simulink model "IntroductiontoSubsystems"  (R2025a)
settings: Solver=VariableStepAuto  StartTime=0.0  StopTime=10.0  RelTol=1e-3
model workspace (MAT data in the model file):
  Ts = 0.01
  ki = 7.33
  kp = 9.39
undefined symbols (not defined in the file or in its folder): b, J, K, L, R, V
libraries: SignalEditorBlockLib x1
settings Model: Creator=JPIRES3  LastModifiedBy=JPIRES3

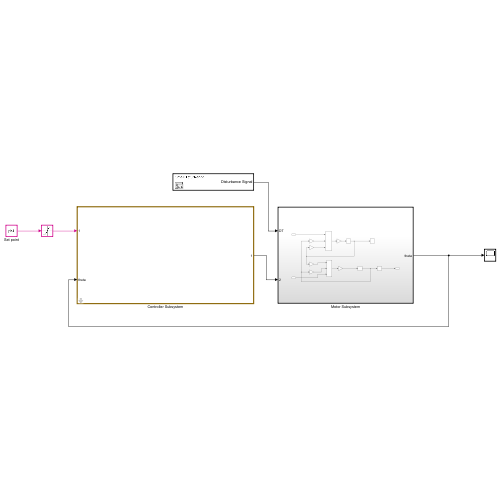
[thumbnail: Simulink's stored preview of the top-level diagram]
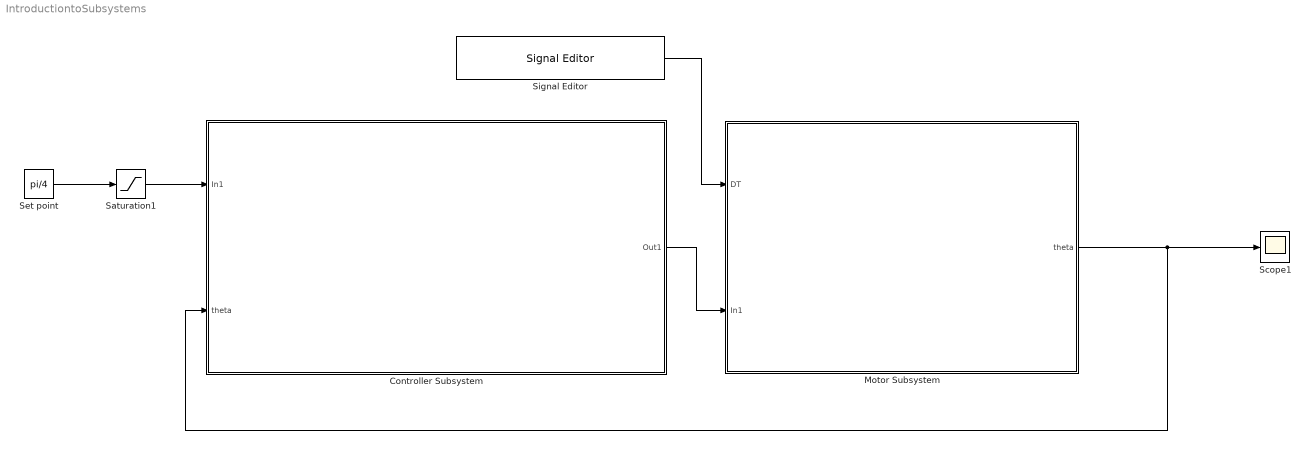
== system IntroductiontoSubsystems ==
  Controller Subsystem : Subsystem  TreatAsAtomicUnit=on  mask{kp=9.39, ki=7.33, Ts=0.01}
      mask prompts: kp "proportional Gain"; ki "Integral Gain"; Ts "Sample Time"
  Motor Subsystem : Subsystem
  Saturation1 : Saturate  UpperLimit=pi/4  LowerLimit=-pi/4
  Scope1 : Scope
      settings: ActiveDisplayYMinimum=-0.11554258584712604  ActiveDisplayYMaximum=1.0398832726241345
  Set point : Constant  Value=pi/4
  Signal Editor : SignalEditorBlockLib/Signal Editor  FileName=C:\Users\jpires3\Documents\Matlab-projects\Module 3 - Introduction to subsystems\Disturbance.mat  ActiveScenario=SmallDisturbance  ActiveSignal=Disturbance Signal  IsBus=off  OutputBusObjectStr=Bus: BusObject  SampleTime=0  ZeroCross=off  OutputAfterFinalValue=Setting to zero  Unit=inherit  PreserveSignalName=on  ApplySigPropsToAllScenarios=on  ApplySigPropsToAllSignals=off  SignalPropertySource=Dialog parameters
  wires:
  Set point/1 -> Saturation1/1
  Motor Subsystem/1(theta) -> Controller Subsystem/2(theta), Scope1/1
  Saturation1/1 -> Controller Subsystem/1(In1)
  Controller Subsystem/1(Out1) -> Motor Subsystem/2(In1)
  Signal Editor/1 -> Motor Subsystem/1(DT)

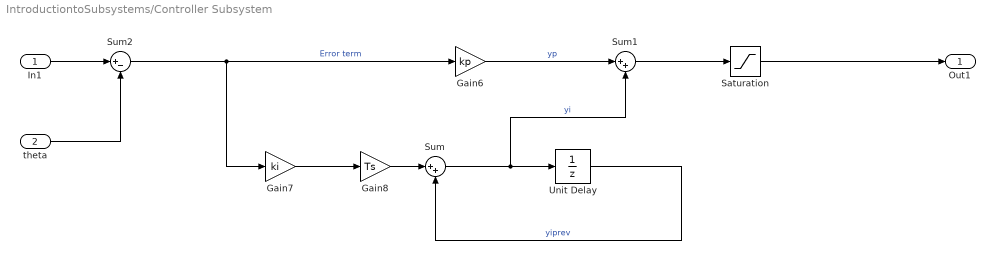
== system IntroductiontoSubsystems/Controller Subsystem ==
  In1 : Inport
  theta : Inport  Port=2
  Gain6 : Gain  Gain=kp
  Gain7 : Gain  Gain=ki
  Gain8 : Gain  Gain=Ts
  Saturation : Saturate  UpperLimit=V  LowerLimit=-V
  Sum : Sum  Inputs=|++
  Sum1 : Sum  Inputs=|++
  Sum2 : Sum  Inputs=|+-
  Unit Delay : UnitDelay  InitialCondition=1  SampleTime=Ts  HasFrameUpgradeWarning=on
  Out1 : Outport
  wires:
  Gain8/1 -> Sum/1
  Sum/1 -> Sum1/2, Unit Delay/1  "yi"
  Sum1/1 -> Saturation/1
  Unit Delay/1 -> Sum/2  "yiprev"
  In1/1 -> Sum2/1
  Gain6/1 -> Sum1/1  "yp"
  Sum2/1 -> Gain7/1, Gain6/1  "Error term"
  Saturation/1 -> Out1/1
  Gain7/1 -> Gain8/1
  theta/1 -> Sum2/2

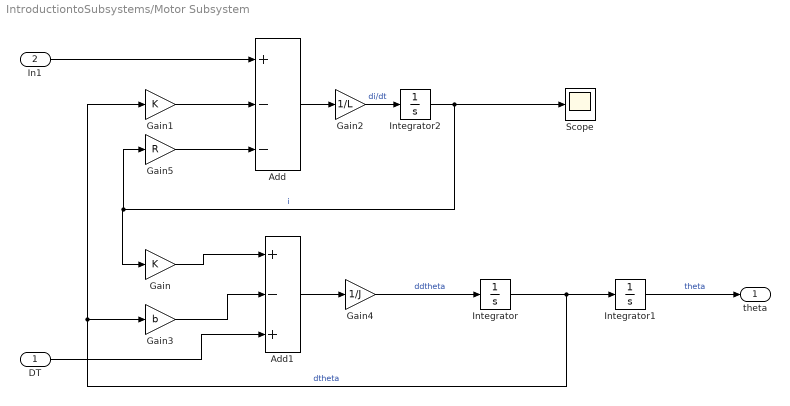
== system IntroductiontoSubsystems/Motor Subsystem ==
  DT : Inport
  In1 : Inport  Port=2
  Add : Sum  Inputs=+--
  Add1 : Sum  Inputs=+-+
  Gain : Gain  Gain=K
  Gain1 : Gain  Gain=K
  Gain2 : Gain  Gain=1/L
  Gain3 : Gain  Gain=b
  Gain4 : Gain  Gain=1/J
  Gain5 : Gain  Gain=R
  Integrator : Integrator
  Integrator1 : Integrator
  Integrator2 : Integrator
  Scope : Scope
      settings: ActiveDisplayYMinimum=-0.073405567669839467  ActiveDisplayYMaximum=0.031632687357691952
  theta : Outport
  wires:
  Integrator/1 -> Integrator1/1, Gain1/1, Gain3/1  "dtheta"
  Gain5/1 -> Add/3
  Add1/1 -> Gain4/1
  Gain1/1 -> Add/2
  Gain3/1 -> Add1/2
  Gain4/1 -> Integrator/1  "ddtheta"
  Gain/1 -> Add1/1
  Integrator2/1 -> Scope/1, Gain5/1, Gain/1  "i"
  Add/1 -> Gain2/1
  Gain2/1 -> Integrator2/1  "di/dt"
  Integrator1/1 -> theta/1  "theta"
  In1/1 -> Add/1
  DT/1 -> Add1/3
